simulink model "richardkinect_modified_2"  (R2012b)
settings: Solver=ode4  StartTime=0.0  StopTime=inf  FixedStep=sample_time  RelTol=1e-3
InitFcn:
  | sample_time=0.005;%0.004;%0.0025;%0.02;
  | sample_time_Vicon = 0.005;
  | DeltaT = 0.02;
  | g = 9.81;
  | H0 = g%0.3165;
  | Kl = 1;
  | 
  | Omega_r = 1.5;%for Horizontal reference
  | Zeta_r = 1; %for Horizontal reference
  | Omega = 1.5;%1.31;%for Horizontal Control
  | Zeta = 0.5;    %for Horizontal Control
  | 
  | Omega_h_r = 2.2; %for vertical reference
  | Zeta_h_r = 1;  %for vertical reference
  | Omega_h = 2.2;    %for vertical control
  | Zeta_h = 1;         %for vertical control
  | PI=pi;
  | 
  | Mass = 0.85;
  | Acc_Max = 4;
  | Acc_Max_h = 4;
  | 
  | Max_RP = 60;
  | 
  | % for NN
  | n = 5;
  | r = 3;
  | n2 = 5;
  | NN_ST = 0.02;
  | 
  | GAMA_V = 3;
  | gama_V_e = 0.01;
  | 
  | GAMA_W = GAMA_V;
  | gama_W_e =0.01;
  | 
  | % deadzone
  | NN_Deadzone_Z = 0;
  | 
  | % inputs nomalizaton parameters
  | NN_Z_y_min = -3;
  | NN_Z_y_max = 0.5;
  | 
  | NN_Z_v_max = 8;
  | NN_Z_v_min = -NN_Z_v_max;
  | 
  | % alpha = 0.034;
  | alpha = 1;
  | % c_f = 0.0015;
  | c_f = 0.001;
  | c_y_tilt = 1*0.5;
  | 
  | %for WK paras
  | Heightcontrol = 0.08;
  | Scale_Factor=1;
  | yoffset=0;
  | 
  | load MaoBi_Oct04_2_int.mat
  | MB_Interp.time = [];
undefined symbols (not defined in the file or in its folder): DiscIntNeverNeededParam
libraries: dspstat3 x6, simulink x5, X330_Control x4, nid_lib x2
settings Model: Creator=ttcl3  LastModifiedBy=Eka
settings SolverCC: MaxConsecutiveMinStep=auto
settings DataIOCC: SignalLoggingSaveFormat=ModelDataLogs
settings DebuggingCC: MultiTaskRateTransMsg=warning  FcnCallInpInsideContextMsg=UseLocalSettings
settings SFSimCC: SimParseCustomCode=off
settings GRTTargetCC: CombineOutputUpdateFcns=off  GRTInterface=on

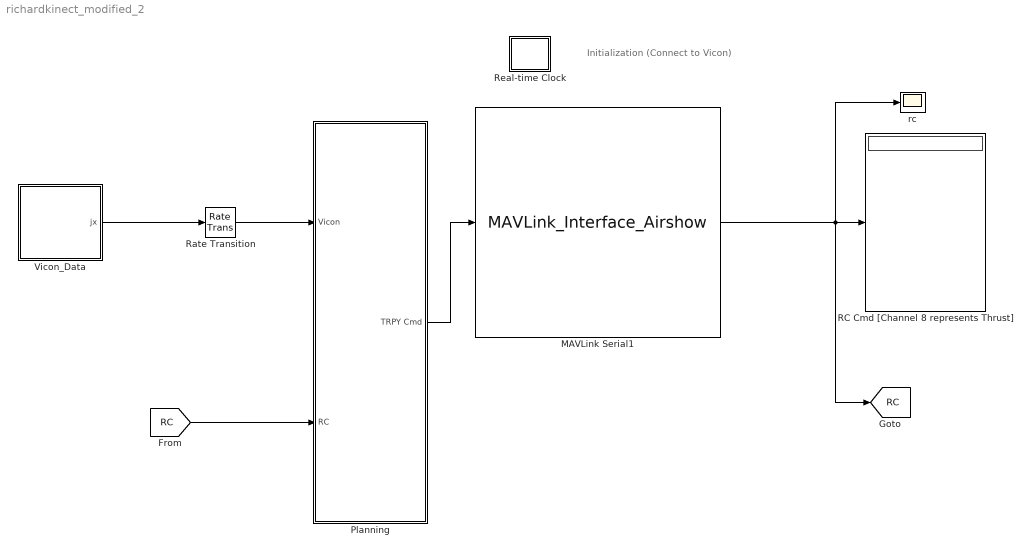
== system richardkinect_modified_2 ==
  note: Initialization
      | (Connect to Vicon)
  MAVLink Serial1 : S-Function  FunctionName=MAVLink_Interface_Airshow  Parameters=COM_Port,Baud_Rate,MSG_INPUT,MSG_OUTPUT  EnableBusSupport=off  mask{COM_Port='COM9', Baud_Rate=57600, ATTITUDE_OUT=off, RC_SCALED=on, Quads_1=on, Quads_2=off, Quads_3=off, Quads_4=off, Quads_5=off, Quads_6=off}
      mask prompts: COM_Port "COM Port"; Baud_Rate "Baud Rate"; ATTITUDE_OUT "DEBUG"; RC_SCALED "RC CHANNELS SCALED"; Quads_1 "1 Quad"; Quads_2 "2 Quad"; Quads_3 "3 Quad"; Quads_4 "4 Quad"; Quads_5 "5 Quad"; Quads_6 "6 Quad"
      mask init:
      | MSG_ID_NUM_INPUT = [ uint8(221) uint8(222) uint8(223) uint8(224) uint8(225) uint8(226)];
      | MSG_ID_NAME_INPUT = [Quads_1 Quads_2 Quads_3 Quads_4 Quads_5 Quads_6];
      | 
      | MSG_ID_NUM_OUTPUT = [uint8(34) uint8(30)];
      | MSG_ID_NAME_OUTPUT = [RC_SCALED ATTITUDE_OUT ];
      | 
      | idx_input = find(MSG_ID_NAME_INPUT);
      | MSG_INPUT = MSG_ID_NUM_INPUT(idx_input);
      | 
      | idx_output = find(MSG_ID_NAME_OUTPUT);
      | MSG_OUTPUT = MSG_ID_NUM_OUTPUT(idx_output);
      mask Display:
      | % Block image
      | image(imread('10-inch Quad Heat Map.png'));
      | 
      | %Label block
      | fprintf('MAVLink Serial\n%s\n%dbps', COM_Port,  Baud_Rate)
      | 
      | 
      | %Label input ports
      | 
      | in = 1;
      | if (Quads_1 == 1)
      |     port_label('input', in, 'Quads_1');
      |     in = in + 1;
      | end
      | 
      | if (Quads_2 == 1)
      |     port_label('input', in, 'Quads_2');
      |     in = in + 1;
      | end
      | 
      | if (Quads_3 == 1)
      |     port_label('input', in, 'Quads_3');
      |     in = in + 1;
      | end
      | 
      | if (Quads_4 == 1)
      |     port_label('input', in, 'Quads_4');
      |     in = in + 1;
      | end
      | 
      | if (Quads_5 == 1)
      |     port_label('input', in, 'Quads_5');
      |     in = in + 1;
      | end
      | 
      | 
      | if (Quads_6 == 1)
      |     port_label('input', in, 'Quads_6');
      |     in = in + 1;
      | end
      | %Label output ports
      | 
      | out = 1;
      | if (RC_SCALED == 1)
      |     port_label('output', out, 'RC CMD');
      |     out = out + 1;
      | end
      | 
      | if (ATTITUDE_OUT == 1)
      |     port_label('output', out, 'DEBUG');
      |     out = out + 1;
      | end
  Planning : Subsystem
  RC Cmd [Channel 8 represents Thrust] : Display
  Rate Transition : RateTransition  OutPortSampleTime=0.02
  Real-time Clock : Subsystem  mask(Real-time Clock){sample_time=0.02, tolerance=1}
      mask prompts: sample_time "Synchronize with real-time every n seconds:"; tolerance "Real-time warning tolerance (seconds):"
      mask help: Real-time Synchronization Block
      mask Help: This block synchronizes simulation time with the PC real-time clock or UNIX system clock. The first dialog entry is the period at which the clock is checked to insure real-time synchronization. The second dialog entry is the number of seconds that the simulation time must be within real-time before a warning is printed.
      mask Display: plot(0,0,100,100,[40,60,60,54,54,64,69,76,82,77,81,83,83,81,78,74,70,64,57,49,41,35,32,30,30,31,34,40,47,47,40,40],[90,90,85,85,80,79,76,87,80,70,64,57,49,41,33,28,24,22,21,23,25,31,37,46,56,65,73,78,80,85,85,90],[69,53,53],[64,50,73])
  Vicon_Data : Subsystem
  rc : Scope
      settings: TimeRange=10  YMin=-1  YMax=0.1
  tag scope: RC=global
  wires:
  [RC] -> Planning/2(RC)
  MAVLink Serial1/1 -> [RC], rc/1, RC Cmd [Channel 8 represents Thrust]/1
  Rate Transition/1 -> Planning/1(Vicon)
  Planning/1(TRPY Cmd) -> MAVLink Serial1/1
  Vicon_Data/1(jx) -> Rate Transition/1

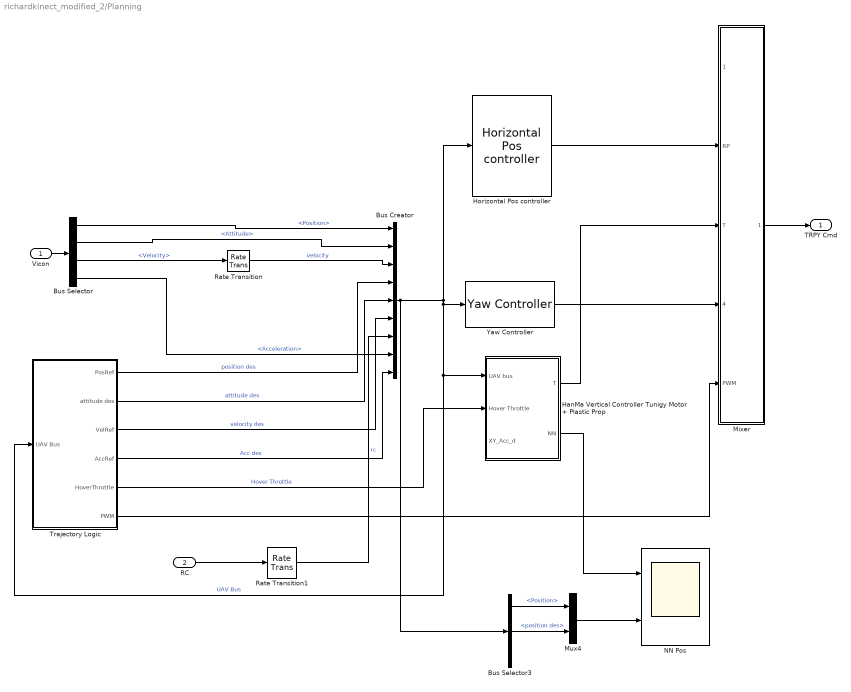
== system richardkinect_modified_2/Planning ==
  Vicon : Inport
  RC : Inport  Port=2
  Bus Creator : BusCreator  Inputs=9
  Bus Selector : BusSelector  OutputSignals=Position,Attitude,Velocity,Acceleration
  Bus Selector3 : BusSelector  OutputSignals=Position,position des,Attitude
  HanMa Vertical Controller Tunigy Motor + Plastic Prop : Subsystem  mask{Omega_h=Omega_h, Zeta_h=Zeta_h, PID_I_h=2, mass=0.85}
      mask prompts: Omega_h "Omega (P Gain  = Omega^2)"; Zeta_h "Zeta (D Gain = 2*Omega*Zeta)"; PID_I_h "I Gain"
  Horizontal Pos controller : X330_Control/Horizontal Pos controller  Max_RP=Max_RP  Omega=Omega  PID_i=0.5  Zeta=Zeta
      link override Horizontal Position Controller/Saturation1: UpperLimit=3.4  LowerLimit=-3.4
  Mixer : Subsystem
  Mux4 : Mux  Inputs=2
  NN Pos : Scope  NumInputPorts=2
      settings: ShowLegends=on  TimeRange=90  YMin=-3~-1.05  YMax=6.5~0.05  SaveName=ScopeData3
  Rate Transition : RateTransition  OutPortSampleTime=0.02
  Rate Transition1 : RateTransition  OutPortSampleTime=0.02
  Trajectory Logic : Subsystem
  Yaw Controller : X330_Control/Yaw Controller
  TRPY Cmd : Outport
  wires:
  Horizontal Pos controller/1 -> Mixer/2(RP)
  Rate Transition/1 -> Bus Creator/3  "velocity"
  Rate Transition1/1 -> Bus Creator/7  "rc"
  Bus Creator/1 -> Yaw Controller/1, Trajectory Logic/1(UAV Bus), HanMa Vertical Controller Tunigy Motor + Plastic Prop/1(UAV bus), Horizontal Pos controller/1, Bus Selector3/1  "UAV Bus"
  Yaw Controller/1 -> Mixer/4(Yaw rate)
  HanMa Vertical Controller Tunigy Motor + Plastic Prop/1(T) -> Mixer/3(T)
  Bus Selector/4 -> Bus Creator/8  "<Acceleration>"
  Trajectory Logic/1(PosRef) -> Bus Creator/4  "position des"
  Trajectory Logic/2(attitude des) -> Bus Creator/5  "attitude des"
  Trajectory Logic/3(VelRef) -> Bus Creator/6  "velocity des"
  Trajectory Logic/5(HoverThrottle) -> HanMa Vertical Controller Tunigy Motor + Plastic Prop/2(Hover Throttle)  "Hover Throttle"
  Bus Selector/1 -> Bus Creator/1  "<Position>"
  Bus Selector/2 -> Bus Creator/2  "<Attitude>"
  Bus Selector/3 -> Rate Transition/1  "<Velocity>"
  Vicon/1 -> Bus Selector/1
  Mixer/1(XYZ RPY) -> TRPY Cmd/1
  Trajectory Logic/4(AccRef) -> Bus Creator/9  "Acc des"
  RC/1 -> Rate Transition1/1
  Trajectory Logic/6(PWM) -> Mixer/5(PWM)
  Mux4/1 -> NN Pos/2
  Bus Selector3/1 -> Mux4/1  "<Position>"
  Bus Selector3/2 -> Mux4/2  "<position des>"
  HanMa Vertical Controller Tunigy Motor + Plastic Prop/2(NN) -> NN Pos/1

== system richardkinect_modified_2/Real-time Clock ==
  Real-time Clock : S-Function  FunctionName=rtclock  Parameters=sample_time, tolerance  EnableBusSupport=off

== system richardkinect_modified_2/Vicon_Data ==
  note: Process Vicon Raw Data to take care of signal loss and object local axis flip
  Constant : Constant
  Logic to fix signal loss and object local axis flip7 : M-S-Function  FunctionName=Vicon_Filter
  Mux22 : Mux  Inputs=2
  Raw Quad Pose from Vicon : Subsystem
  Transfer Fcn : TransferFcn  Denominator=[1 1]
  Vicon Filter : X330_Control/Vicon Filter
  jx : Outport
  wires:
  Raw Quad Pose from Vicon/2(Attitude_Vicon_jx) -> Mux22/2
  Raw Quad Pose from Vicon/1(Position_Vicon_jx) -> Mux22/1
  Logic to fix signal loss and object local axis flip7/1 -> Vicon Filter/1
  Constant/1 -> Transfer Fcn/1
  Mux22/1 -> Logic to fix signal loss and object local axis flip7/1
  Vicon Filter/1 -> jx/1

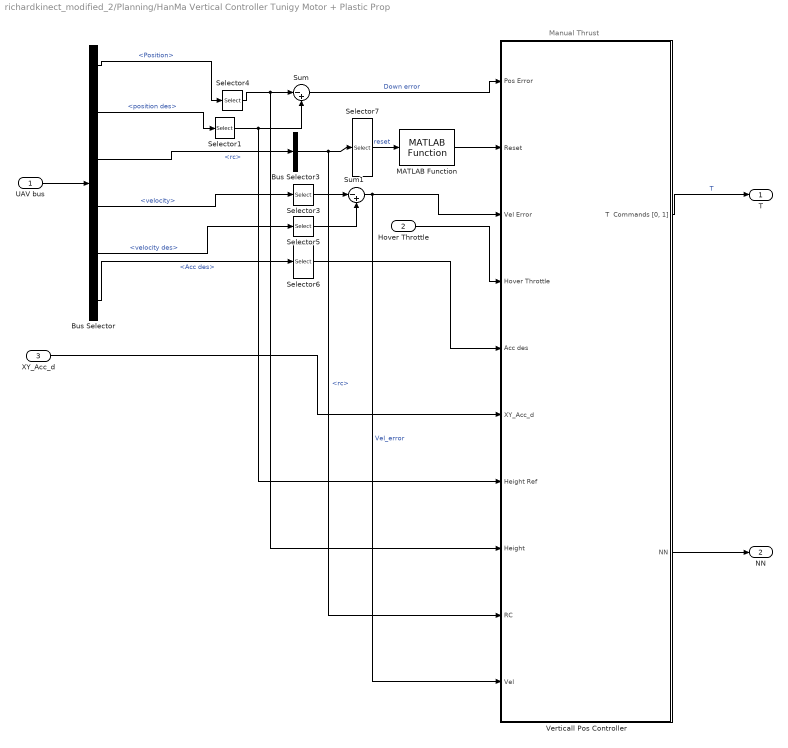
== system richardkinect_modified_2/Planning/HanMa Vertical Controller Tunigy Motor + Plastic Prop ==
  note: Manual Thrust
  UAV bus : Inport
  Hover Throttle : Inport  Port=2
  XY_Acc_d : Inport  Port=3
  Bus Selector : BusSelector  OutputSignals=Position,position des,rc,velocity,velocity des,Acc des
  Bus Selector3 : BusSelector  OutputSignals=rc
  MATLAB Function : X330_Control/NN For Height AxiMotor + APC Prop/MATLAB Function
  Selector{1,3..5} (4 alike) : Selector  InputPortWidth=3  IndexOptions=Index vector (dialog)  Indices=[3]  OutputSizes=1
  Selector6 : Selector  InputPortWidth=4  IndexOptions=Index vector (dialog)  Indices=[3]  OutputSizes=1
  Selector7 : Selector  InputPortWidth=8  IndexOptions=Index vector (dialog)  Indices=[7]  OutputSizes=1
  Sum : Sum  Inputs=|-+
  Sum1 : Sum  Inputs=|-+
  Verticall Pos Controller : Subsystem
  T : Outport
  NN : Outport  Port=2
  wires:
  XY_Acc_d/1 -> Verticall Pos Controller/6(XY_Acc_d)
  Verticall Pos Controller/1("T  Commands [0, 1]") -> T/1  "T"
  Selector6/1 -> Verticall Pos Controller/5(Acc des)
  Bus Selector/6 -> Selector6/1  "<Acc des>"
  Hover Throttle/1 -> Verticall Pos Controller/4(Hover Throttle)
  Bus Selector/5 -> Selector5/1  "<velocity des>"
  Bus Selector/4 -> Selector3/1  "<velocity>"
  Selector5/1 -> Sum1/2
  Selector3/1 -> Sum1/1
  Sum1/1 -> Verticall Pos Controller/3(Vel Error), Verticall Pos Controller/10(Vel)  "Vel_error"
  Selector7/1 -> MATLAB Function/1  "reset"
  Bus Selector3/1 -> Selector7/1, Verticall Pos Controller/9(RC)  "<rc>"
  Selector1/1 -> Sum/2, Verticall Pos Controller/7(Height Ref)
  Selector4/1 -> Sum/1, Verticall Pos Controller/8(Height)
  Sum/1 -> Verticall Pos Controller/1(Pos Error)  "Down error"
  Bus Selector/2 -> Selector1/1  "<position des>"
  Bus Selector/1 -> Selector4/1  "<Position>"
  Bus Selector/3 -> Bus Selector3/1  "<rc>"
  UAV bus/1 -> Bus Selector/1
  Verticall Pos Controller/2(NN) -> NN/1
  MATLAB Function/1 -> Verticall Pos Controller/2(Reset)

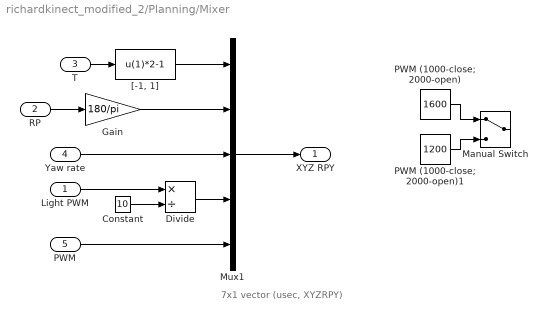
== system richardkinect_modified_2/Planning/Mixer ==
  note: 7x1 vector (usec, XYZRPY)
  Light PWM : Inport
  RP : Inport  Port=2
  T : Inport  Port=3
  Yaw rate : Inport  Port=4
  PWM : Inport  Port=5
  Constant : Constant  Value=10
  Divide : Product  Inputs=*/
  Gain : Gain  Gain=180/pi
  Manual Switch : ManualSwitch
  Mux1 : Mux  Inputs=5
  PWM (1000-close; 2000-open) : Constant  Value=1600  SampleTime=0.02
  PWM (1000-close; 2000-open)1 : Constant  Value=1200  SampleTime=0.02
  "[-1, 1]" : Fcn  Expr=u(1)*2-1
  XYZ RPY : Outport
  wires:
  Mux1/1 -> XYZ RPY/1
  T/1 -> "[-1, 1]"/1
  RP/1 -> Gain/1
  PWM (1000-close; 2000-open)/1 -> Manual Switch/1
  PWM (1000-close; 2000-open)1/1 -> Manual Switch/2
  Gain/1 -> Mux1/2
  "[-1, 1]"/1 -> Mux1/1
  PWM/1 -> Mux1/5
  Constant/1 -> Divide/2
  Yaw rate/1 -> Mux1/3
  Divide/1 -> Mux1/4
  Light PWM/1 -> Divide/1

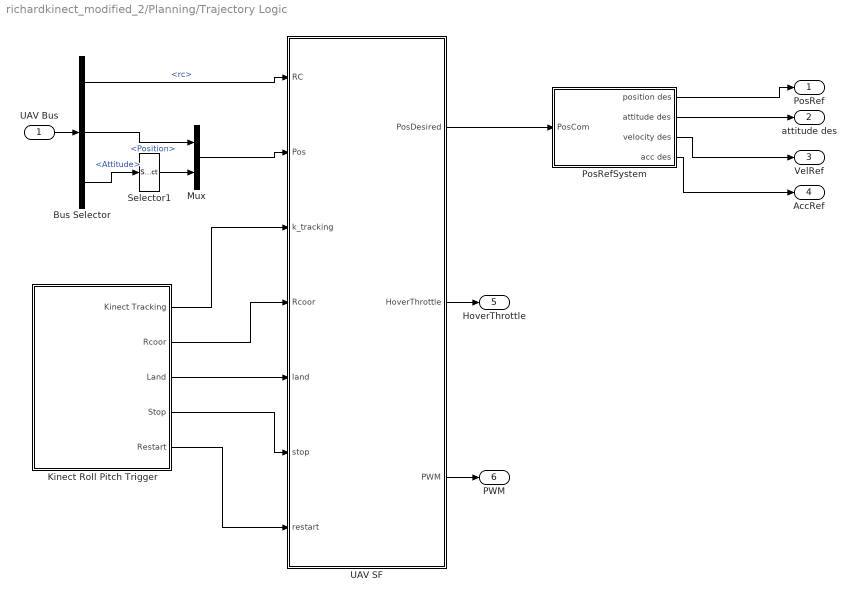
== system richardkinect_modified_2/Planning/Trajectory Logic ==
  UAV Bus : Inport
  Bus Selector : BusSelector  OutputSignals=rc,Position,Attitude
  Kinect Roll Pitch Trigger : Subsystem
  Mux : Mux  Inputs=2
  PosRefSystem : Subsystem  AncestorBlock=X330_Control/PosRefSystem  mask{Omega_r=Omega_r, Zeta_r=Zeta_r, Acc_Max=Acc_Max, Omega_h_r=Omega_h_r, Zeta_h_r=Zeta_h_r, Acc_h_Max=Acc_Max_h}
      mask prompts: Omega_r "Omega_r (P Gain= Omega_r^2)"; Zeta_r "Zeta_r (D = 2*Omega_r*Zeta_r)"
  Selector1 : Selector  InputPortWidth=3  IndexOptions=Index vector (dialog)  Indices=[3]  OutputSizes=1
  UAV SF : Stateflow chart  TreatAsAtomicUnit=on
  PosRef : Outport
  attitude des : Outport  Port=2
  VelRef : Outport  Port=3
  AccRef : Outport  Port=4
  HoverThrottle : Outport  Port=5
  PWM : Outport  Port=6
  wires:
  UAV SF/1(PosDesired) -> PosRefSystem/1(PosCom)
  Bus Selector/1 -> UAV SF/1(RC)  "<rc>"
  UAV SF/2(HoverThrottle) -> HoverThrottle/1
  UAV Bus/1 -> Bus Selector/1
  Bus Selector/2 -> Mux/1  "<Position>"
  Bus Selector/3 -> Selector1/1  "<Attitude>"
  Selector1/1 -> Mux/2
  Mux/1 -> UAV SF/2(Pos)
  UAV SF/3(PWM) -> PWM/1
  PosRefSystem/1(position des) -> PosRef/1
  PosRefSystem/3(velocity des) -> VelRef/1
  PosRefSystem/4(acc des) -> AccRef/1
  PosRefSystem/2(attitude des) -> attitude des/1
  Kinect Roll Pitch Trigger/1(Kinect Tracking) -> UAV SF/3(k_tracking)
  Kinect Roll Pitch Trigger/2(Rcoor) -> UAV SF/4(Rcoor)
  Kinect Roll Pitch Trigger/3(Land) -> UAV SF/5(land)
  Kinect Roll Pitch Trigger/4(Stop) -> UAV SF/6(stop)
  Kinect Roll Pitch Trigger/5(Restart) -> UAV SF/7(restart)

== system richardkinect_modified_2/Vicon_Data/Raw Quad Pose from Vicon ==
  Constant : Constant
  Demux : Demux  Outputs=1
  Interpreted MATLAB Function : MATLABFcn  MATLABFcn=Kinect20140120  SampleTime=0.005
  Process Vicon Raw Data7 : Subsystem
  Position_Vicon_jx : Outport
  Attitude_Vicon_jx : Outport  Port=2
  wires:
  Process Vicon Raw Data7/1(Position) -> Position_Vicon_jx/1
  Process Vicon Raw Data7/2(Attitude) -> Attitude_Vicon_jx/1
  Constant/1 -> Interpreted MATLAB Function/1
  Interpreted MATLAB Function/1 -> Demux/1
  Demux/1 -> Process Vicon Raw Data7/1(Vicon Raw)

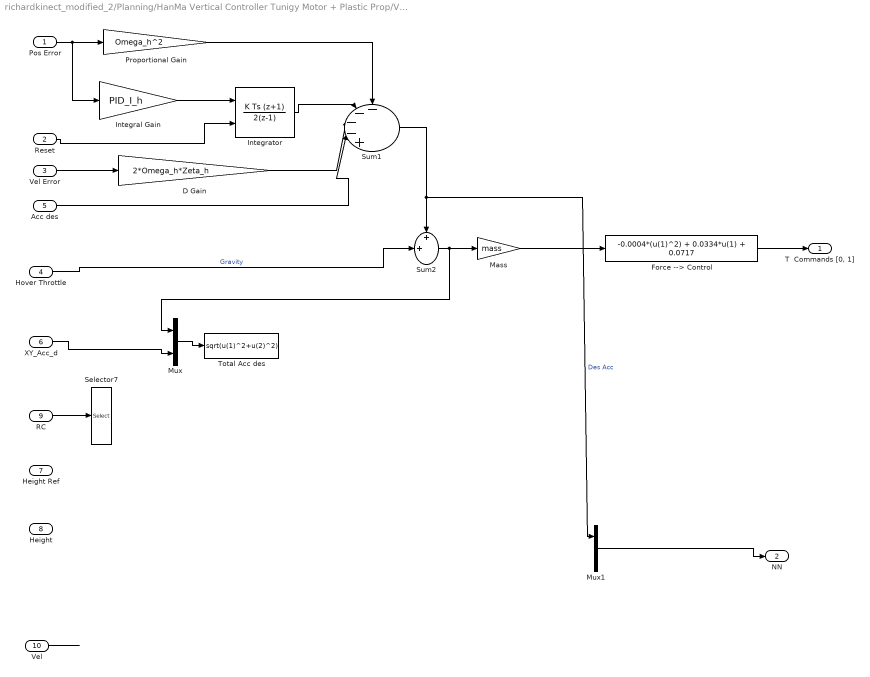
== system richardkinect_modified_2/Planning/HanMa Vertical Controller Tunigy Motor + Plastic Prop/Verticall Pos Controller ==
  Pos Error : Inport
  Reset : Inport  Port=2
  Vel Error : Inport  Port=3
  Hover Throttle : Inport  Port=4
  Acc des : Inport  Port=5
  XY_Acc_d : Inport  Port=6
  Height Ref : Inport  Port=7
  Height : Inport  Port=8
  RC : Inport  Port=9
  Vel : Inport  Port=10
  D Gain : Gain  Gain=2*Omega_h*Zeta_h  OutDataTypeStr=double
  Force --> Control : Fcn  Expr=-0.0004*(u(1)^2) + 0.0334*u(1) + 0.0717
  Integral Gain : Gain  DisableCoverage=on  Gain=PID_I_h  ParamDataTypeStr=double  OutDataTypeStr=double
  Integrator : DiscreteIntegrator  DisableCoverage=on  IntegratorMethod=Integration: Trapezoidal  ExternalReset=level  InitialConditionMode=State only (most efficient)  SampleTime=-1  OutDataTypeStr=double  UpperSaturationLimit=0.3  LowerSaturationLimit=-0.3  ICPrevOutput=DiscIntNeverNeededParam  ICPrevScaledInput=DiscIntNeverNeededParam
  Mass : Gain  DisableCoverage=on  Gain=mass  ParamDataTypeStr=double  OutDataTypeStr=double
  Mux : Mux  Inputs=2
  Mux1 : Mux  Inputs=2
  Proportional Gain : Gain  DisableCoverage=on  Gain=Omega_h^2  ParamDataTypeStr=double  OutDataTypeStr=double
  Selector7 : Selector  InputPortWidth=8  IndexOptions=Index vector (dialog)  Indices=[6]  OutputSizes=1
  Sum1 : Sum  DisableCoverage=on  Inputs=----+|  AccumDataTypeStr=double  OutDataTypeStr=double  SampleTime=0.02
  Sum2 : Sum  DisableCoverage=on  Inputs=++|  AccumDataTypeStr=double  OutDataTypeStr=double  SampleTime=0.02
  Total Acc des : Fcn  Expr=sqrt(u(1)^2+u(2)^2)
  "T  Commands [0, 1]" : Outport
  NN : Outport  Port=2
  wires:
  Force --> Control/1 -> "T  Commands [0, 1]"/1
  Sum2/1 -> Mux/1, Mass/1
  XY_Acc_d/1 -> Mux/2
  Mux/1 -> Total Acc des/1
  Mass/1 -> Force --> Control/1
  Sum1/1 -> Sum2/1, Mux1/1  "Des Acc"
  Hover Throttle/1 -> Sum2/2  "Gravity"
  Acc des/1 -> Sum1/4
  D Gain/1 -> Sum1/3
  Vel Error/1 -> D Gain/1
  Reset/1 -> Integrator/2
  Pos Error/1 -> Integral Gain/1, Proportional Gain/1
  Proportional Gain/1 -> Sum1/1
  Integrator/1 -> Sum1/2
  Integral Gain/1 -> Integrator/1
  RC/1 -> Selector7/1
  Mux1/1 -> NN/1
  Vel/1 -> ?

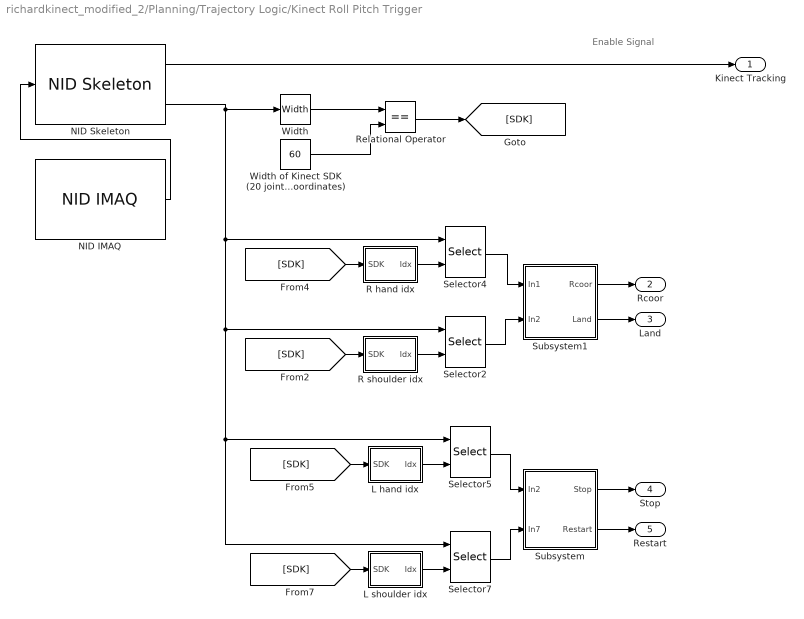
== system richardkinect_modified_2/Planning/Trajectory Logic/Kinect Roll Pitch Trigger ==
  note: Enable Signal
  L hand idx : Subsystem
  L shoulder idx : Subsystem
  NID IMAQ : nid_lib/NID IMAQ  imaq_depth=off  imaq_motion=off  imaq_image=off  view_point=off  imaq_skeleton=on  imaq_ir=off  mirror_image=off  imaq_sample_time=1/25  res_fps=VGA (640x480): 30 FPS  needPsiPose=off  angle_input=off  angle=0  angle_read=off  near_mode=off  seated_mode=on  skeleton_smooth=[1.0 0.5 0.5 0.05 0.04]  infer_skeleton=on
  NID Skeleton : nid_lib/NID Skeleton  num_of_skeleton_tracking=1  conv_XYZ_RW=on  viewer=off
  R hand idx : Subsystem
  R shoulder idx : Subsystem
  Relational Operator : RelationalOperator  Operator===  OutDataTypeStr=boolean
  Selector{2,4..5,7} (4 alike) : Selector  NumberOfDimensions=3  InputPortWidth=3  IndexOptions=Select all,Index vector (port),Select all  Indices=[1 3],1,1  OutputSizes=1,1,1
  Subsystem : Subsystem
  Subsystem1 : Subsystem
  Width : Width
  Width of Kinect SDK (20 joints x 3 coordinates) : Constant  Value=60
  Kinect Tracking : Outport
  Rcoor : Outport  Port=2
  Land : Outport  Port=3
  Stop : Outport  Port=4
  Restart : Outport  Port=5
  wires:
  [SDK] -> R hand idx/1(SDK)
  R hand idx/1(Idx) -> Selector4/2
  [SDK] -> R shoulder idx/1(SDK)
  R shoulder idx/1(Idx) -> Selector2/2
  NID Skeleton/1 -> Kinect Tracking/1
  Relational Operator/1 -> [SDK]
  Width of Kinect SDK (20 joints x 3 coordinates)/1 -> Relational Operator/2
  Width/1 -> Relational Operator/1
  NID IMAQ/1 -> NID Skeleton/1
  [SDK] -> L hand idx/1(SDK)
  [SDK] -> L shoulder idx/1(SDK)
  L hand idx/1(Idx) -> Selector5/2
  L shoulder idx/1(Idx) -> Selector7/2
  NID Skeleton/2 -> Selector7/1, Selector5/1, Selector2/1, Selector4/1, Width/1
  Selector4/1 -> Subsystem1/1(In1)
  Selector2/1 -> Subsystem1/2(In2)
  Selector5/1 -> Subsystem/1(In2)
  Selector7/1 -> Subsystem/2(In7)
  Subsystem/1(Stop) -> Stop/1
  Subsystem/2(Restart) -> Restart/1
  Subsystem1/1(Rcoor) -> Rcoor/1
  Subsystem1/2(Land) -> Land/1

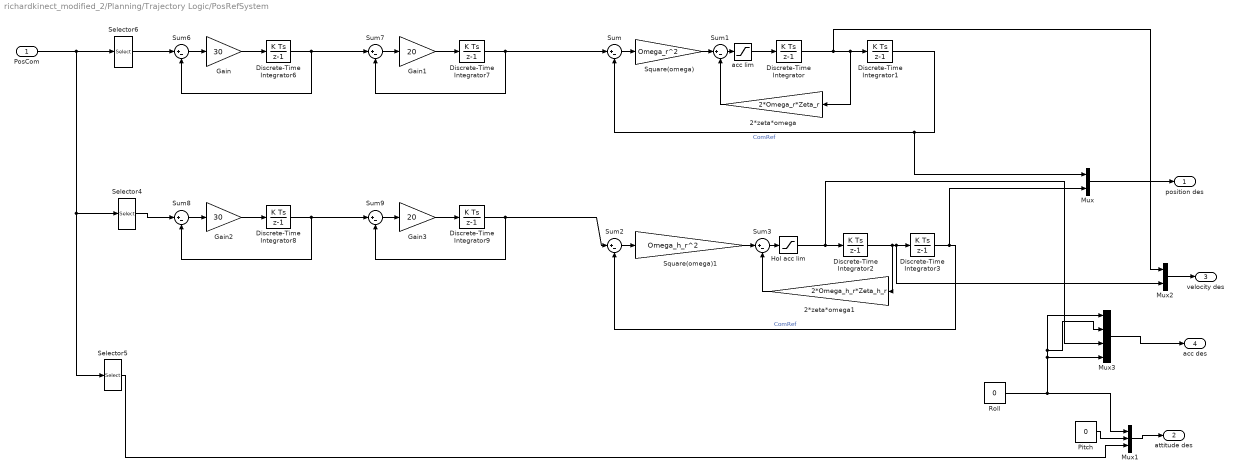
== system richardkinect_modified_2/Planning/Trajectory Logic/PosRefSystem ==
  PosCom : Inport
  2*zeta*omega : Gain  Gain=2*Omega_r*Zeta_r
  2*zeta*omega1 : Gain  Gain=2*Omega_h_r*Zeta_h_r
  Discrete-Time Integrator{,1..3,6..9} (8 alike) : DiscreteIntegrator  SampleTime=-1  ICPrevOutput=DiscIntNeverNeededParam  ICPrevScaledInput=DiscIntNeverNeededParam
  Gain : Gain  Gain=30
  Gain1 : Gain  Gain=20
  Gain2 : Gain  Gain=30
  Gain3 : Gain  Gain=20
  Hol acc lim : Saturate  UpperLimit=Acc_h_Max  LowerLimit=-Acc_h_Max
  Mux : Mux  Inputs=2
  Mux1 : Mux  Inputs=3
  Mux2 : Mux  Inputs=2
  Mux3 : Mux
  Pitch : Constant  Value=0  SampleTime=0.02
  Roll : Constant  Value=0  SampleTime=0.02
  Selector4 : Selector  InputPortWidth=4  IndexOptions=Index vector (dialog)  Indices=[3]  OutputSizes=1
  Selector5 : Selector  InputPortWidth=4  IndexOptions=Index vector (dialog)  Indices=[4]  OutputSizes=1
  Selector6 : Selector  InputPortWidth=4  IndexOptions=Index vector (dialog)  Indices=[1 2]  OutputSizes=1
  Square(omega) : Gain  Gain=Omega_r^2
  Square(omega)1 : Gain  Gain=Omega_h_r^2
  Sum{,1..3,6..9} (8 alike) : Sum  Inputs=|+-
  acc lim : Saturate  UpperLimit=Acc_Max  LowerLimit=-Acc_Max
  position des : Outport
  attitude des : Outport  Port=2
  velocity des : Outport  Port=3
  acc des : Outport  Port=4
  wires:
  Sum9/1 -> Gain3/1
  Gain3/1 -> Discrete-Time Integrator9/1
  Discrete-Time Integrator9/1 -> Sum2/1, Sum9/2
  Sum8/1 -> Gain2/1
  Gain2/1 -> Discrete-Time Integrator8/1
  Discrete-Time Integrator8/1 -> Sum9/1, Sum8/2
  Selector4/1 -> Sum8/1
  Sum7/1 -> Gain1/1
  Gain1/1 -> Discrete-Time Integrator7/1
  Discrete-Time Integrator7/1 -> Sum/1, Sum7/2
  Sum6/1 -> Gain/1
  Gain/1 -> Discrete-Time Integrator6/1
  Discrete-Time Integrator6/1 -> Sum7/1, Sum6/2
  Selector6/1 -> Sum6/1
  Mux3/1 -> acc des/1
  Mux2/1 -> velocity des/1
  Mux1/1 -> attitude des/1
  Pitch/1 -> Mux1/2
  Mux/1 -> position des/1
  Discrete-Time Integrator1/1 -> Mux/1, Sum/2  "ComRef"
  Hol acc lim/1 -> Mux3/3, Discrete-Time Integrator2/1
  2*zeta*omega1/1 -> Sum3/2
  Sum3/1 -> Hol acc lim/1
  Discrete-Time Integrator2/1 -> Mux2/2, Discrete-Time Integrator3/1, 2*zeta*omega1/1
  Square(omega)1/1 -> Sum3/1
  Sum2/1 -> Square(omega)1/1
  Discrete-Time Integrator3/1 -> Mux/2, Sum2/2  "ComRef"
  acc lim/1 -> Discrete-Time Integrator/1
  2*zeta*omega/1 -> Sum1/2
  Sum1/1 -> acc lim/1
  Discrete-Time Integrator/1 -> Mux2/1, 2*zeta*omega/1, Discrete-Time Integrator1/1
  Square(omega)/1 -> Sum1/1
  Sum/1 -> Square(omega)/1
  PosCom/1 -> Selector6/1, Selector5/1, Selector4/1
  Selector5/1 -> Mux1/3
  Roll/1 -> Mux3/2, Mux3/1, Mux3/4, Mux1/1

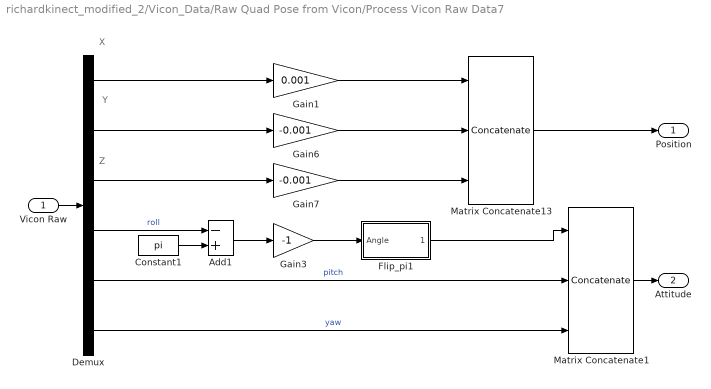
== system richardkinect_modified_2/Vicon_Data/Raw Quad Pose from Vicon/Process Vicon Raw Data7 ==
  note: X
  note: Y
  note: Z
  Vicon Raw : Inport
  Add1 : Sum  Inputs=-+
  Constant1 : Constant  Value=pi  OutDataTypeStr=double
  Demux : Demux  Outputs=6
  Flip_pi1 : Subsystem  mask(Flip -pi to pi){}
      mask help: Flips the inputs into the range -pi to pi
      mask Help: Flips the inputs into the range -pi to pi
      mask Display: disp('Flip_pi')
  Gain1 : Gain  Gain=0.001
  Gain3 : Gain  Gain=-1
  Gain6 : Gain  Gain=-0.001
  Gain7 : Gain  Gain=-0.001
  Matrix Concatenate1 : Concatenate  NumInputs=3  Mode=Multidimensional array
  Matrix Concatenate13 : Concatenate  NumInputs=3  Mode=Multidimensional array
  Position : Outport
  Attitude : Outport  Port=2
  wires:
  Constant1/1 -> Add1/2
  Demux/6 -> Matrix Concatenate1/3  "yaw"
  Gain1/1 -> Matrix Concatenate13/1
  Demux/1 -> Gain1/1
  Demux/2 -> Gain6/1
  Demux/3 -> Gain7/1
  Demux/4 -> Add1/1  "roll"
  Gain6/1 -> Matrix Concatenate13/2
  Gain7/1 -> Matrix Concatenate13/3
  Add1/1 -> Gain3/1
  Gain3/1 -> Flip_pi1/1(Angle)
  Demux/5 -> Matrix Concatenate1/2  "pitch"
  Flip_pi1/1(Angle_Flip) -> Matrix Concatenate1/1
  Matrix Concatenate13/1 -> Position/1
  Vicon Raw/1 -> Demux/1
  Matrix Concatenate1/1 -> Attitude/1

== system richardkinect_modified_2/Planning/Trajectory Logic/Kinect Roll Pitch Trigger/L hand idx ==
  SDK : Inport
  Kinect SDK : Constant  Value=8
  OpenNI : Constant  Value=9
  Switch : Switch  Criteria=u2 ~= 0
  Idx : Outport
  wires:
  Kinect SDK/1 -> Switch/1
  OpenNI/1 -> Switch/3
  SDK/1 -> Switch/2
  Switch/1 -> Idx/1

== system richardkinect_modified_2/Planning/Trajectory Logic/Kinect Roll Pitch Trigger/L shoulder idx ==
  SDK : Inport
  Kinect SDK : Constant  Value=5
  OpenNI : Constant  Value=7
  Switch : Switch  Criteria=u2 ~= 0
  Idx : Outport
  wires:
  Kinect SDK/1 -> Switch/1
  OpenNI/1 -> Switch/3
  SDK/1 -> Switch/2
  Switch/1 -> Idx/1

== system richardkinect_modified_2/Planning/Trajectory Logic/Kinect Roll Pitch Trigger/R hand idx ==
  SDK : Inport
  Kinect SDK : Constant  Value=12
  OpenNI : Constant  Value=6
  Switch : Switch  Criteria=u2 ~= 0
  Idx : Outport
  wires:
  Switch/1 -> Idx/1
  SDK/1 -> Switch/2
  OpenNI/1 -> Switch/3
  Kinect SDK/1 -> Switch/1

== system richardkinect_modified_2/Planning/Trajectory Logic/Kinect Roll Pitch Trigger/R shoulder idx ==
  SDK : Inport
  Kinect SDK : Constant  Value=9
  OpenNI : Constant  Value=4
  Switch : Switch  Criteria=u2 ~= 0
  Idx : Outport
  wires:
  Switch/1 -> Idx/1
  SDK/1 -> Switch/2
  OpenNI/1 -> Switch/3
  Kinect SDK/1 -> Switch/1

== system richardkinect_modified_2/Planning/Trajectory Logic/Kinect Roll Pitch Trigger/Subsystem ==
  In2 : Inport
  In7 : Inport  Port=2
  Start : simulink/Logic and Bit Operations/Compare To Constant  relop=>=  const=0.3  OutDataTypeStr=uint8
  Stp : simulink/Logic and Bit Operations/Compare To Constant  relop=>=  const=0.4  OutDataTypeStr=boolean
  Subtract : Subsystem
  XYZtoX_Y_Z2 : Subsystem
  XYZtoX_Y_Z4 : Subsystem
  Stop : Outport
  Restart : Outport  Port=2
  wires:
  In2/1 -> XYZtoX_Y_Z2/1(XYZ)
  In7/1 -> XYZtoX_Y_Z4/1(XYZ)
  XYZtoX_Y_Z2/1(X) -> Subtract/1(In1)
  XYZtoX_Y_Z2/2(Y) -> Subtract/2(In2)
  XYZtoX_Y_Z2/3(Z) -> Subtract/3(In3)
  XYZtoX_Y_Z4/1(X) -> Subtract/4(In4)
  XYZtoX_Y_Z4/2(Y) -> Subtract/5(In5)
  XYZtoX_Y_Z4/3(Z) -> Subtract/6(In6)
  Subtract/1(x_coor) -> Stp/1
  Stp/1 -> Stop/1
  Start/1 -> Restart/1
  Subtract/2(y_coor) -> Start/1

== system richardkinect_modified_2/Planning/Trajectory Logic/Kinect Roll Pitch Trigger/Subsystem1 ==
  In1 : Inport
  In2 : Inport  Port=2
  Compare To Constant : simulink/Logic and Bit Operations/Compare To Constant  relop=<=  const=0.3  OutDataTypeStr=uint8
  Mapping : Subsystem
  Subtract : Subsystem
  XYZtoX_Y_Z1 : Subsystem
  XYZtoX_Y_Z3 : Subsystem
  Rcoor : Outport
  Land : Outport  Port=2
  wires:
  In1/1 -> XYZtoX_Y_Z1/1(XYZ)
  In2/1 -> XYZtoX_Y_Z3/1(XYZ)
  XYZtoX_Y_Z1/1(X) -> Subtract/1(In1)
  XYZtoX_Y_Z1/2(Y) -> Subtract/2(In2)
  XYZtoX_Y_Z1/3(Z) -> Subtract/3(In3)
  XYZtoX_Y_Z3/1(X) -> Subtract/4(In4)
  XYZtoX_Y_Z3/2(Y) -> Subtract/5(In5)
  XYZtoX_Y_Z3/3(Z) -> Subtract/6(In6)
  Subtract/1(x_coor) -> Mapping/1(x_coor)
  Subtract/2(y_coor) -> Mapping/2(y_coor)
  Subtract/3(z_coor) -> Compare To Constant/1, Mapping/3(z_coor)
  Mapping/1(Rcoor) -> Rcoor/1
  Compare To Constant/1 -> Land/1

== system richardkinect_modified_2/Vicon_Data/Raw Quad Pose from Vicon/Process Vicon Raw Data7/Flip_pi1 ==
  Angle : Inport
  Add : Sum  Inputs=-+
  Compare To Constant1 : simulink/Logic and Bit Operations/Compare To Constant  relop=>  const=pi  OutDataTypeStr=uint8  ZeroCross=off
  Constant : Constant  Value=2*pi
  Data Type Duplicate : DataTypeDuplicate
  Flip_0_to_2pi : Subsystem  mask(Flip zero to 2pi){}
      mask help: Flips the inputs into the range zero to +2pi
      mask Help: Flips the inputs into the range zero to +2pi
      mask Display: disp('Flip_0_2pi')
  Switch : Switch  Criteria=u2 ~= 0
  Angle_Flip : Outport
  wires:
  Switch/1 -> Data Type Duplicate/1, Angle_Flip/1
  Add/1 -> Switch/1
  Constant/1 -> Add/1
  Compare To Constant1/1 -> Switch/2
  Flip_0_to_2pi/1(Angle_Flip) -> Add/2, Compare To Constant1/1, Switch/3
  Angle/1 -> Data Type Duplicate/2, Flip_0_to_2pi/1(Angle)

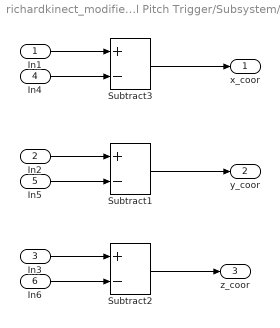
== system richardkinect_modified_2/Planning/Trajectory Logic/Kinect Roll Pitch Trigger/Subsystem/Subtract ==
  In1 : Inport
  In2 : Inport  Port=2
  In3 : Inport  Port=3
  In4 : Inport  Port=4
  In5 : Inport  Port=5
  In6 : Inport  Port=6
  Subtract1 : Sum  Inputs=+-
  Subtract2 : Sum  Inputs=+-
  Subtract3 : Sum  Inputs=+-
  x_coor : Outport
  y_coor : Outport  Port=2
  z_coor : Outport  Port=3
  wires:
  In1/1 -> Subtract3/1
  In2/1 -> Subtract1/1
  In3/1 -> Subtract2/1
  In4/1 -> Subtract3/2
  In5/1 -> Subtract1/2
  In6/1 -> Subtract2/2
  Subtract2/1 -> z_coor/1
  Subtract1/1 -> y_coor/1
  Subtract3/1 -> x_coor/1

== system richardkinect_modified_2/Planning/Trajectory Logic/Kinect Roll Pitch Trigger/Subsystem/XYZtoX_Y_Z2 ==
  XYZ : Inport
  Selector : Selector  NumberOfDimensions=3  InputPortWidth=3  IndexOptions=Index vector (dialog),Index vector (dialog),Index vector (dialog)  Indices=1,1,1  OutputSizes=1,1,1
  Selector1 : Selector  NumberOfDimensions=3  InputPortWidth=3  IndexOptions=Index vector (dialog),Index vector (dialog),Index vector (dialog)  Indices=1,1,2  OutputSizes=1,1,1
  Selector2 : Selector  NumberOfDimensions=3  InputPortWidth=3  IndexOptions=Index vector (dialog),Index vector (dialog),Index vector (dialog)  Indices=1,1,3  OutputSizes=1,1,1
  X : Outport
  Y : Outport  Port=2
  Z : Outport  Port=3
  wires:
  XYZ/1 -> Selector/1, Selector1/1, Selector2/1
  Selector/1 -> X/1
  Selector1/1 -> Y/1
  Selector2/1 -> Z/1

== system richardkinect_modified_2/Planning/Trajectory Logic/Kinect Roll Pitch Trigger/Subsystem/XYZtoX_Y_Z4 ==
  XYZ : Inport
  Selector : Selector  NumberOfDimensions=3  InputPortWidth=3  IndexOptions=Index vector (dialog),Index vector (dialog),Index vector (dialog)  Indices=1,1,1  OutputSizes=1,1,1
  Selector1 : Selector  NumberOfDimensions=3  InputPortWidth=3  IndexOptions=Index vector (dialog),Index vector (dialog),Index vector (dialog)  Indices=1,1,2  OutputSizes=1,1,1
  Selector2 : Selector  NumberOfDimensions=3  InputPortWidth=3  IndexOptions=Index vector (dialog),Index vector (dialog),Index vector (dialog)  Indices=1,1,3  OutputSizes=1,1,1
  X : Outport
  Y : Outport  Port=2
  Z : Outport  Port=3
  wires:
  Selector2/1 -> Z/1
  Selector1/1 -> Y/1
  Selector/1 -> X/1
  XYZ/1 -> Selector2/1, Selector1/1, Selector/1

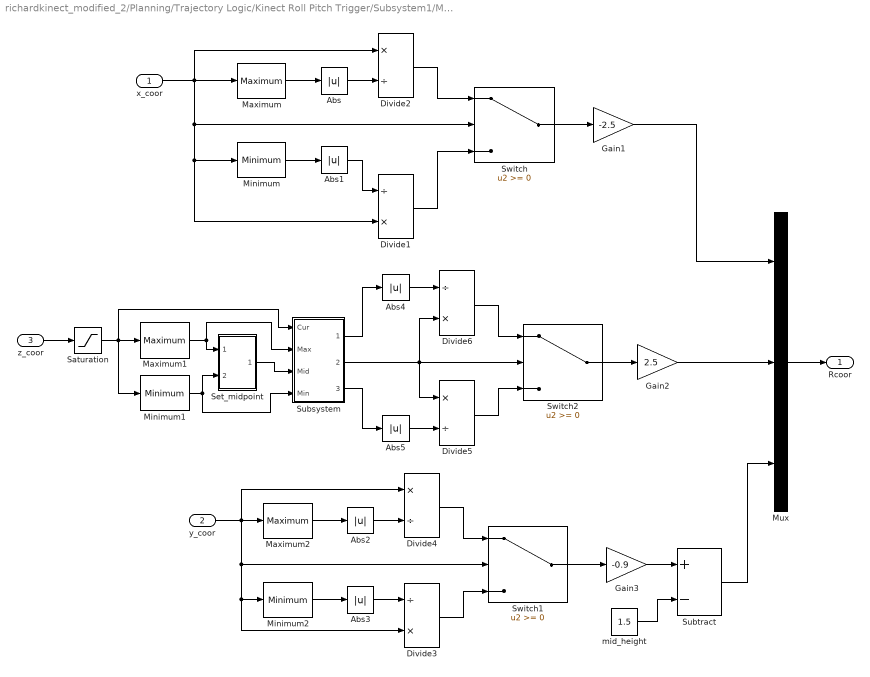
== system richardkinect_modified_2/Planning/Trajectory Logic/Kinect Roll Pitch Trigger/Subsystem1/Mapping ==
  x_coor : Inport
  y_coor : Inport  Port=2
  z_coor : Inport  Port=3
  Abs{,1..5} (6 alike) : Abs
  Divide1 : Product  Inputs=/*
  Divide2 : Product  Inputs=*/
  Divide3 : Product  Inputs=/*
  Divide4 : Product  Inputs=*/
  Divide5 : Product  Inputs=*/
  Divide6 : Product  Inputs=/*
  Gain1 : Gain  Gain=-2.5
  Gain2 : Gain  Gain=2.5
  Gain3 : Gain  Gain=-0.9
  Maximum : dspstat3/Maximum  fcn=Running  reset=None  indexBase=One  operateOver=Each column  Dimension=1  colComp=on  operation=maximum  roiEnable=off  roiType=Rectangles  roiPortion=Entire ROI  roiOutput=Individual statistics for each ROI  roiFlag=off  accumDataTypeStr=Inherit: Same as product output  accumLastDataTypeStr=Inherit: Same as product output  roundingMode=Floor  overflowMode=off
  Maximum1 : dspstat3/Maximum  fcn=Running  reset=None  indexBase=One  operateOver=Each column  Dimension=1  colComp=on  operation=maximum  roiEnable=off  roiType=Rectangles  roiPortion=Entire ROI  roiOutput=Individual statistics for each ROI  roiFlag=off  accumDataTypeStr=Inherit: Same as product output  accumLastDataTypeStr=Inherit: Same as product output  roundingMode=Floor  overflowMode=off
  Maximum2 : dspstat3/Maximum  fcn=Running  reset=None  indexBase=One  operateOver=Each column  Dimension=1  colComp=on  operation=maximum  roiEnable=off  roiType=Rectangles  roiPortion=Entire ROI  roiOutput=Individual statistics for each ROI  roiFlag=off  accumDataTypeStr=Inherit: Same as product output  accumLastDataTypeStr=Inherit: Same as product output  roundingMode=Floor  overflowMode=off
  Minimum : dspstat3/Minimum  fcn=Running  reset=None  indexBase=One  operateOver=Each column  Dimension=1  colComp=on  operation=minimum  roiEnable=off  roiType=Rectangles  roiPortion=Entire ROI  roiOutput=Individual statistics for each ROI  roiFlag=off  roundingMode=Floor  overflowMode=off
  Minimum1 : dspstat3/Minimum  fcn=Running  reset=None  indexBase=One  operateOver=Each column  Dimension=1  colComp=on  operation=minimum  roiEnable=off  roiType=Rectangles  roiPortion=Entire ROI  roiOutput=Individual statistics for each ROI  roiFlag=off  roundingMode=Floor  overflowMode=off
  Minimum2 : dspstat3/Minimum  fcn=Running  reset=None  indexBase=One  operateOver=Each column  Dimension=1  colComp=on  operation=minimum  roiEnable=off  roiType=Rectangles  roiPortion=Entire ROI  roiOutput=Individual statistics for each ROI  roiFlag=off  roundingMode=Floor  overflowMode=off
  Mux : Mux  Inputs=3
  Saturation : Saturate  UpperLimit=-0.15  LowerLimit=-4
  Set_midpoint : Subsystem
  Subsystem : Subsystem
  Subtract : Sum  Inputs=+-
  Switch : Switch
  Switch1 : Switch
  Switch2 : Switch
  mid_height : Constant  Value=1.5
  Rcoor : Outport
  wires:
  Minimum/1 -> Abs1/1
  Abs/1 -> Divide2/2
  Divide2/1 -> Switch/1
  Abs1/1 -> Divide1/1
  Divide1/1 -> Switch/3
  Switch/1 -> Gain1/1
  y_coor/1 -> Maximum2/1, Minimum2/1, Divide3/2, Switch1/2, Divide4/1
  Minimum2/1 -> Abs3/1
  Abs2/1 -> Divide4/2
  Divide4/1 -> Switch1/1
  Abs3/1 -> Divide3/1
  Divide3/1 -> Switch1/3
  Divide6/1 -> Switch2/1
  Divide5/1 -> Switch2/3
  z_coor/1 -> Saturation/1
  Switch2/1 -> Gain2/1
  Mux/1 -> Rcoor/1
  Gain1/1 -> Mux/1
  Maximum/1 -> Abs/1
  x_coor/1 -> Maximum/1, Divide2/1, Switch/2, Minimum/1, Divide1/2
  Maximum2/1 -> Abs2/1
  Maximum1/1 -> Subsystem/2(Max), Set_midpoint/1(max)
  Minimum1/1 -> Subsystem/4(Min), Set_midpoint/2(min)
  Abs4/1 -> Divide6/1
  Abs5/1 -> Divide5/2
  Gain2/1 -> Mux/2
  Subsystem/2(curref) -> Divide6/2, Divide5/1, Switch2/2
  Subsystem/1(maxabs) -> Abs4/1
  Subsystem/3(minabs) -> Abs5/1
  Set_midpoint/1(Mid) -> Subsystem/3(Mid)
  Switch1/1 -> Gain3/1
  Subtract/1 -> Mux/3
  mid_height/1 -> Subtract/2
  Gain3/1 -> Subtract/1
  Saturation/1 -> Minimum1/1, Subsystem/1(Cur), Maximum1/1

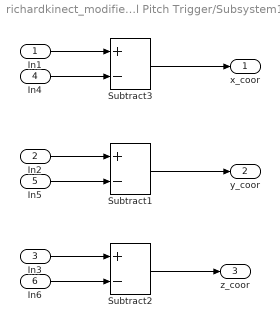
== system richardkinect_modified_2/Planning/Trajectory Logic/Kinect Roll Pitch Trigger/Subsystem1/Subtract ==
  In1 : Inport
  In2 : Inport  Port=2
  In3 : Inport  Port=3
  In4 : Inport  Port=4
  In5 : Inport  Port=5
  In6 : Inport  Port=6
  Subtract1 : Sum  Inputs=+-
  Subtract2 : Sum  Inputs=+-
  Subtract3 : Sum  Inputs=+-
  x_coor : Outport
  y_coor : Outport  Port=2
  z_coor : Outport  Port=3
  wires:
  In1/1 -> Subtract3/1
  In2/1 -> Subtract1/1
  In3/1 -> Subtract2/1
  In4/1 -> Subtract3/2
  In5/1 -> Subtract1/2
  In6/1 -> Subtract2/2
  Subtract2/1 -> z_coor/1
  Subtract1/1 -> y_coor/1
  Subtract3/1 -> x_coor/1

== system richardkinect_modified_2/Planning/Trajectory Logic/Kinect Roll Pitch Trigger/Subsystem1/XYZtoX_Y_Z1 ==
  XYZ : Inport
  Selector : Selector  NumberOfDimensions=3  InputPortWidth=3  IndexOptions=Index vector (dialog),Index vector (dialog),Index vector (dialog)  Indices=1,1,1  OutputSizes=1,1,1
  Selector1 : Selector  NumberOfDimensions=3  InputPortWidth=3  IndexOptions=Index vector (dialog),Index vector (dialog),Index vector (dialog)  Indices=1,1,2  OutputSizes=1,1,1
  Selector2 : Selector  NumberOfDimensions=3  InputPortWidth=3  IndexOptions=Index vector (dialog),Index vector (dialog),Index vector (dialog)  Indices=1,1,3  OutputSizes=1,1,1
  X : Outport
  Y : Outport  Port=2
  Z : Outport  Port=3
  wires:
  Selector2/1 -> Z/1
  Selector1/1 -> Y/1
  Selector/1 -> X/1
  XYZ/1 -> Selector2/1, Selector1/1, Selector/1

== system richardkinect_modified_2/Planning/Trajectory Logic/Kinect Roll Pitch Trigger/Subsystem1/XYZtoX_Y_Z3 ==
  XYZ : Inport
  Selector : Selector  NumberOfDimensions=3  InputPortWidth=3  IndexOptions=Index vector (dialog),Index vector (dialog),Index vector (dialog)  Indices=1,1,1  OutputSizes=1,1,1
  Selector1 : Selector  NumberOfDimensions=3  InputPortWidth=3  IndexOptions=Index vector (dialog),Index vector (dialog),Index vector (dialog)  Indices=1,1,2  OutputSizes=1,1,1
  Selector2 : Selector  NumberOfDimensions=3  InputPortWidth=3  IndexOptions=Index vector (dialog),Index vector (dialog),Index vector (dialog)  Indices=1,1,3  OutputSizes=1,1,1
  X : Outport
  Y : Outport  Port=2
  Z : Outport  Port=3
  wires:
  XYZ/1 -> Selector/1, Selector1/1, Selector2/1
  Selector/1 -> X/1
  Selector1/1 -> Y/1
  Selector2/1 -> Z/1

== system richardkinect_modified_2/Vicon_Data/Raw Quad Pose from Vicon/Process Vicon Raw Data7/Flip_pi1/Flip_0_to_2pi ==
  Angle : Inport
  Add : Sum
  Compare To Constant1 : simulink/Logic and Bit Operations/Compare To Constant  relop=<  const=0  OutDataTypeStr=uint8  ZeroCross=off
  Constant : Constant  Value=2*pi
  Data Type Duplicate : DataTypeDuplicate
  Flip_2pi : Subsystem  mask(Flip -2pi to 2pi){}
      mask help: Flips the inputs into the range -2pi to +2pi
      mask Help: Flips the inputs into the range -2pi to +2pi
      mask Display: disp('Flip_2pi')
  Switch : Switch  Criteria=u2 ~= 0
  Angle_Flip : Outport
  wires:
  Switch/1 -> Data Type Duplicate/1, Angle_Flip/1
  Angle/1 -> Data Type Duplicate/2, Flip_2pi/1(Angle)
  Add/1 -> Switch/1
  Constant/1 -> Add/1
  Compare To Constant1/1 -> Switch/2
  Flip_2pi/1(Angle_Flip) -> Switch/3, Add/2, Compare To Constant1/1

== system richardkinect_modified_2/Planning/Trajectory Logic/Kinect Roll Pitch Trigger/Subsystem1/Mapping/Set_midpoint ==
  max : Inport
  min : Inport  Port=2
  Add : Sum
  Gain : Gain  Gain=0.5
  Mid : Outport
  wires:
  min/1 -> Add/2
  Add/1 -> Gain/1
  Gain/1 -> Mid/1
  max/1 -> Add/1

== system richardkinect_modified_2/Planning/Trajectory Logic/Kinect Roll Pitch Trigger/Subsystem1/Mapping/Subsystem ==
  Cur : Inport
  Max : Inport  Port=2
  Mid : Inport  Port=3
  Min : Inport  Port=4
  Subtract : Sum  Inputs=+-
  Subtract1 : Sum  Inputs=+-
  Subtract2 : Sum  Inputs=+-
  maxabs : Outport
  curref : Outport  Port=2
  minabs : Outport  Port=3
  wires:
  Subtract/1 -> maxabs/1
  Subtract1/1 -> minabs/1
  Subtract2/1 -> curref/1
  Mid/1 -> Subtract1/2, Subtract2/2, Subtract/2
  Cur/1 -> Subtract2/1
  Min/1 -> Subtract1/1
  Max/1 -> Subtract/1

== system richardkinect_modified_2/Vicon_Data/Raw Quad Pose from Vicon/Process Vicon Raw Data7/Flip_pi1/Flip_0_to_2pi/Flip_2pi ==
  Angle : Inport
  Bias : Bias  Bias=-2*pi
  Constant : Constant  Value=2*pi
  Data Type Duplicate : DataTypeDuplicate
  Modulo : Math  Operator=mod  SaturateOnIntegerOverflow=on
  Sign1 : Signum
  Switch : Switch
  Angle_Flip : Outport
  wires:
  Switch/1 -> Data Type Duplicate/2, Angle_Flip/1
  Bias/1 -> Switch/3
  Sign1/1 -> Switch/2
  Modulo/1 -> Switch/1, Bias/1
  Constant/1 -> Modulo/2
  Angle/1 -> Data Type Duplicate/1, Sign1/1, Modulo/1

== stateflow chart richardkinect_modified_2/Planning/Trajectory Logic/UAV SF ==
  state AirBorne
    state Order
      state Stay
        en:
        PosDesired = Pos;
        PosDesired[3] = 0;
      state Projection
        du:
        PosDesired[0] = Rcoor[0];
        PosDesired[1] = Rcoor[1];
        PosDesired[2] = Rcoor[2];
      (default) -> Stay
      Projection -> Stay : [stop == 1]
      Stay -> Projection : [restart == 1]
    state ResetYaw
      en:
      PosDesired = Pos;
      PosDesired[3] = 0;
    state TakeOff
      du:HoverThrottle = (H0 - HoverThrottle)*0.25*DeltaT + HoverThrottle ;
      PosDesired[2] = (-1.2- PosDesired[2])*1*DeltaT + PosDesired[2] ;
    state Landing1
      state Descending
        en:PosDesired = Pos;
        du:PosDesired[2] = (0.2- PosDesired[2])*0.8*DeltaT + PosDesired[2] ;
      state CutThrottle
        en: PWM=1600;
        du:HoverThrottle = (0.0- HoverThrottle)*3*DeltaT + HoverThrottle ;
      (default) -> AirBorne.Landing1.Descending
      AirBorne.Landing1.Descending -> AirBorne.Landing1.CutThrottle : [Pos[2] >(0.0 -0.2)]
    (default) -> TakeOff : {PosDesired = Pos;}
    ResetYaw -> Order : [k_tracking == 1]
    TakeOff -> ResetYaw : after(5,sec)
    Order -> ResetYaw [order 2] : [k_tracking == 0]
    Landing1 -> TakeOff : [restart == 1]
    Order -> Landing1 [order 1] : [land == 1]
  state Landing
    state Descending
      en:PosDesired = Pos;
      du:PosDesired[2] = (0.2- PosDesired[2])*0.8*DeltaT + PosDesired[2] ;
    state CutThrottle
      en: PWM=1600;
      du:HoverThrottle = (0.0- HoverThrottle)*3*DeltaT + HoverThrottle ;
    (default) -> Landing.Descending
    Landing.Descending -> Landing.CutThrottle : [Pos[2] >(0.0 -0.2)]
  Landing -> AirBorne : [RC[6] > 0.5]
  AirBorne -> Landing : [RC[6] < -0.5]
  (default) -> Landing : {HoverThrottle = 0;}
  data: PosDesired output double size=4; HoverThrottle output double size=1; RC input size=8; Pos input size=4; DeltaT parameter size=1; H0 parameter size=1; Kl parameter size=1; VelCmd local double size=2 =0; PWM output double; PI parameter size=1; k_tracking input; Rcoor input; land input; stop input; restart input
